simulink model "THRESHER_CONTROLLER_ROS2"  (R2026a)
settings: Solver=FixedStepAuto  StopTime=inf  FixedStep=0.05  EnableMultiTasking=on
undefined symbols (not defined in the file): C_ph, C_sy, DiscIntNeverNeededParam, GAMMA_ph, GAMMA_sy, K1_ph, K1_sy, K2_ph, K2_sy, L_ph, L_sy, PHI_ph, PHI_sy, T, y, z
libraries: ros2lib x4
settings Model: Creator=The MathWorks, Inc.  LastModifiedBy=env
settings OptimizationCC: PassReuseOutputArgsThreshold=0.0
settings HardwareCC: ProdBitPerLong=64.0  ProdHWDeviceType=Intel->x86-64 (Linux 64)  TargetBitPerLong=64.0  TargetBitPerPointer=64.0  TargetBitPerSizeT=64.0  TargetBitPerPtrDiffT=64.0  TargetLargestAtomicFloat=Float  TargetIntDivRoundTo=Zero  TargetEndianess=LittleEndian  TargetWordSize=64.0  TargetHWDeviceType=Intel->x86-64 (Linux 64)  UseEmbeddedCoderFeatures=off
settings SFSimCC: SimTargetLang=C++
settings RTWCC: SystemTargetFile=ert.tlc  HardwareBoard=Robot Operating System 2 (ROS 2)  TLCOptions="-aInlineSetEventsForThisBaseRateFcn=TLC_FALSE -aSuppressMultiTaskScheduler=TLC_FALSE  -aRateBasedStepFcn=0"  GenCodeOnly=on  Toolchain=Colcon Tools  TargetLang=C++  Description=Embedded Coder
settings ERTTargetCC: ExtModeTransport=2.0  ExtModeAutomaticAllocSize=off  DynamicArrayContainerType=coder::array  ERTCustomFileBanners=off  CodeInterfacePackaging=C++ class  SupportContinuousTime=on  SupportNonInlinedSFcns=on  SupportVariableSizeSignals=on  ModelStepFunctionPrototypeControlCompliant=off

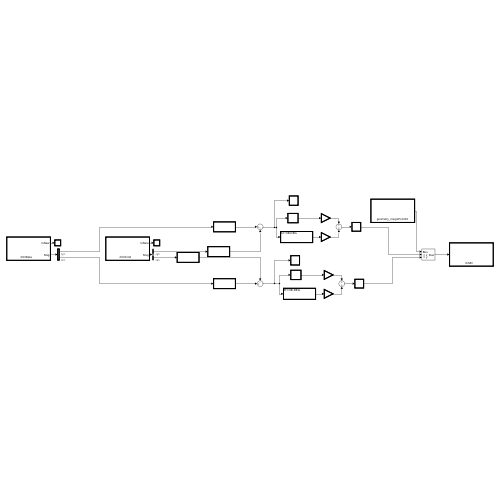
[thumbnail: Simulink's stored preview of the top-level diagram]
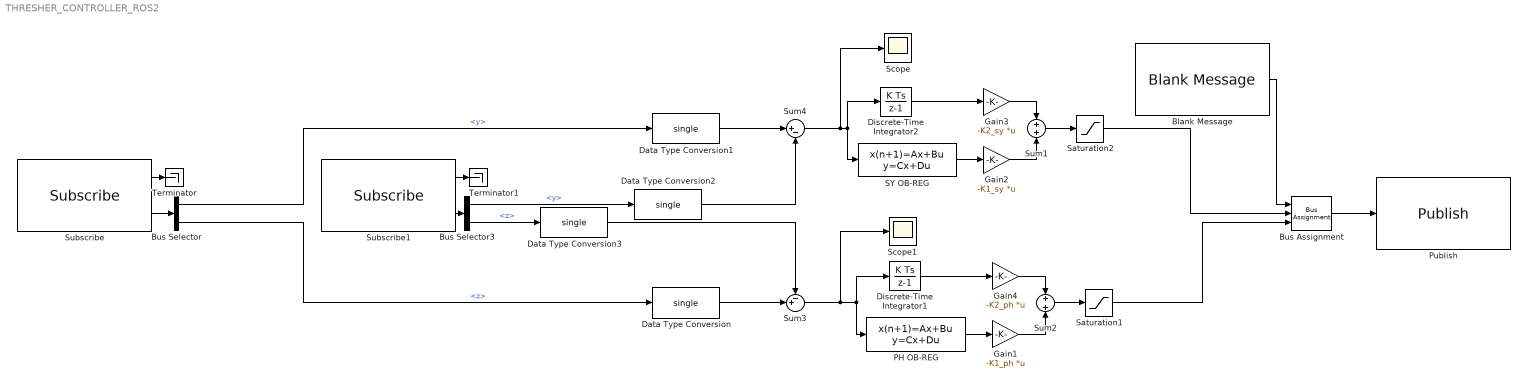
== system THRESHER_CONTROLLER_ROS2 ==
  Blank Message : ros2lib/Blank Message  messageClass=Message  entityType=geometry_msgs/Point32  messageType=geometry_msgs/Point32  SampleTime=inf
  Bus Assignment : BusAssignment  AssignedSignals=z,y
  Bus Selector : BusSelector  OutputSignals=y,z
  Bus Selector3 : BusSelector  OutputSignals=y,z
  Data Type Conversion{,1..3} (4 alike) : DataTypeConversion  OutDataTypeStr=single  SaturateOnIntegerOverflow=off  RndMeth=Floor
  Discrete-Time Integrator1 : DiscreteIntegrator  gainval=1  SampleTime=T  LimitOutput=on  UpperSaturationLimit=(-pi/6)/K2_ph  LowerSaturationLimit=(pi/6)/K2_ph  ICPrevOutput=DiscIntNeverNeededParam  ICPrevScaledInput=DiscIntNeverNeededParam
  Discrete-Time Integrator2 : DiscreteIntegrator  gainval=1  SampleTime=T  LimitOutput=on  UpperSaturationLimit=(pi/6)/K2_sy  LowerSaturationLimit=(-pi/6)/K2_sy  ICPrevOutput=DiscIntNeverNeededParam  ICPrevScaledInput=DiscIntNeverNeededParam
  Gain1 : Gain  Gain=-K1_ph  Multiplication=Matrix(K*u)
  Gain2 : Gain  Gain=-K1_sy  Multiplication=Matrix(K*u)
  Gain3 : Gain  Gain=-K2_sy  Multiplication=Matrix(K*u)
  Gain4 : Gain  Gain=-K2_ph  Multiplication=Matrix(K*u)
  PH OB-REG : DiscreteStateSpace  A=(PHI_ph-L_ph*C_ph-GAMMA_ph*K1_ph)  B=L_ph  C=eye(4)  D=zeros(4,1)  InitialCondition=[0;0;0;0]  SampleTime=T
  Publish : ros2lib/Publish  topicSource=Specify your own  topic=/CMD  messageType=geometry_msgs/Point32  QOSHistory=Keep last  QOSDepth=10  QOSReliability=Reliable  QOSDurability=Volatile  QOSDeadline=Inf  QOSLifespan=Inf  QOSLiveliness=Automatic  QOSLeaseDuration=Inf  QOSAvoidROSNamespaceConventions=off
  SY OB-REG : DiscreteStateSpace  A=(PHI_sy-L_sy*C_sy-GAMMA_sy*K1_sy)  B=L_sy  C=eye(3)  D=zeros(3,1)  InitialCondition=[0;0;0]  SampleTime=T
  Saturation1 : Saturate  UpperLimit=pi/6  LowerLimit=-pi/6
  Saturation2 : Saturate  UpperLimit=pi/6  LowerLimit=-pi/6
  Scope : Scope
      settings: ActiveDisplayYMinimum=-3.5580872401387507  ActiveDisplayYMaximum=0.60685862535082613
  Scope1 : Scope
      settings: ActiveDisplayYMinimum=-29.24533814523306  ActiveDisplayYMaximum=9.7072929322376744
  Subscribe : ros2lib/Subscribe  topicSource=Specify your own  topic=/CtrlData  messageType=geometry_msgs/Point  sampleTime=-1  QOSHistory=Keep last  QOSDepth=10  QOSReliability=Reliable  QOSDurability=Volatile  QOSDeadline=Inf  QOSLifespan=Inf  QOSLiveliness=Automatic  QOSLeaseDuration=Inf  QOSAvoidROSNamespaceConventions=off
  Subscribe1 : ros2lib/Subscribe  topicSource=Specify your own  topic=/CtrlCmd  messageType=geometry_msgs/Point  sampleTime=-1  QOSHistory=Keep last  QOSDepth=10  QOSReliability=Reliable  QOSDurability=Volatile  QOSDeadline=Inf  QOSLifespan=Inf  QOSLiveliness=Automatic  QOSLeaseDuration=Inf  QOSAvoidROSNamespaceConventions=off
  Sum1 : Sum  Inputs=+|+
  Sum2 : Sum  Inputs=+|+
  Sum3 : Sum  Inputs=-+|
  Sum4 : Sum  Inputs=|+-
  Terminator : Terminator
  Terminator1 : Terminator
  wires:
  PH OB-REG/1 -> Gain1/1
  Discrete-Time Integrator1/1 -> Gain4/1
  Gain1/1 -> Sum2/2
  Sum2/1 -> Saturation1/1
  Sum3/1 -> Scope1/1, PH OB-REG/1, Discrete-Time Integrator1/1
  SY OB-REG/1 -> Gain2/1
  Sum4/1 -> Scope/1, SY OB-REG/1, Discrete-Time Integrator2/1
  Sum1/1 -> Saturation2/1
  Discrete-Time Integrator2/1 -> Gain3/1
  Gain2/1 -> Sum1/2
  Gain3/1 -> Sum1/1
  Gain4/1 -> Sum2/1
  Subscribe1/1 -> Terminator1/1
  Bus Assignment/1 -> Publish/1
  Blank Message/1 -> Bus Assignment/1
  Saturation1/1 -> Bus Assignment/3
  Saturation2/1 -> Bus Assignment/2
  Bus Selector/1 -> Data Type Conversion1/1  "<y>"
  Bus Selector/2 -> Data Type Conversion/1  "<z>"
  Subscribe/2 -> Bus Selector/1
  Subscribe/1 -> Terminator/1
  Bus Selector3/1 -> Data Type Conversion2/1  "<y>"
  Subscribe1/2 -> Bus Selector3/1
  Data Type Conversion/1 -> Sum3/2
  Data Type Conversion3/1 -> Sum3/1
  Data Type Conversion2/1 -> Sum4/2
  Data Type Conversion1/1 -> Sum4/1
  Bus Selector3/2 -> Data Type Conversion3/1  "<z>"
